simulink model "closeLoopv2"  (R2024a)
settings: Solver=ode4  StartTime=0.0  StopTime=2000  FixedStep=1E-4  MinStep=1E-4  RelTol=1e-3
values from neighbouring files (symbols this model uses):
  initial_1 =     [ma.mat]    (also in regulation.mat)
  x = [input(1);input(2);input(3)]    [Dist_observer.m]    (also in is501nmtbModel_simu.m; is501nmtbModel_simu1.m; ma.mat = ; neuronalPID.m = entr(4))
  y = [input(7),input(8),input(9)]'    [estimator.m]    (also in is501nmtbModel_simu.m = B * x; is501nmtbModel_simu1.m = B * x + Td; ma.mat = ; regulation.mat = )
  z =     [ma.mat]    (also in regulation.mat)
settings Model: Creator=b_ant  LastModifiedBy=b_ant
settings SolverCC: InitialStep=1E-4  ZeroCrossAlgorithm=Adaptive
settings DebuggingCC: IgnoredZcDiagnostic=none

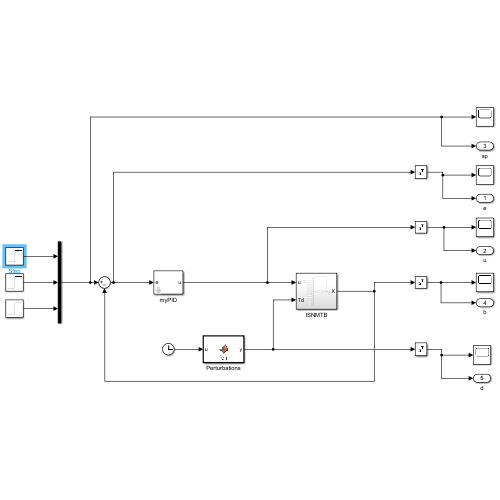
[thumbnail: Simulink's stored preview of the top-level diagram]
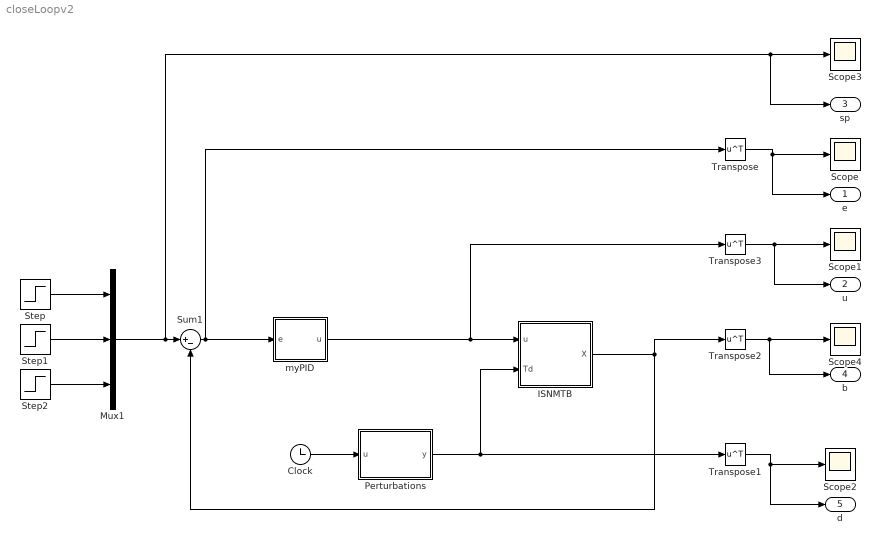
== system closeLoopv2 ==
  Clock : Clock
      settings: Decimation=1000
  ISNMTB : Subsystem
  Mux1 : Mux  Inputs=3
  Perturbations : MATLAB Function  TreatAsAtomicUnit=on
  Scope{,1..4} (5 alike) : Scope
  Step : Step  Time=0.1  After=0  SampleTime=0
  Step1 : Step  Time=0.1  After=0  SampleTime=0
  Step2 : Step  Time=0.1  After=0  SampleTime=0
  Sum1 : Sum  Inputs=|+-
  Transpose{,1..3} (4 alike) : Math  Operator=transpose
  myPID : Subsystem
  e : Outport
  u : Outport  Port=2
  sp : Outport  Port=3
  b : Outport  Port=4
  d : Outport  Port=5
  wires:
  Step2/1 -> Mux1/3
  Sum1/1 -> myPID/1(e), Transpose/1
  Step1/1 -> Mux1/2
  Perturbations/1(y) -> Transpose1/1, ISNMTB/2(Td)
  Clock/1 -> Perturbations/1(u)
  Step/1 -> Mux1/1
  Transpose/1 -> e/1, Scope/1
  Transpose1/1 -> Scope2/1, d/1
  ISNMTB/1(X) -> Transpose2/1, Sum1/2
  Transpose2/1 -> b/1, Scope4/1
  Transpose3/1 -> u/1, Scope1/1
  Mux1/1 -> sp/1, Scope3/1, Sum1/1
  myPID/1(u) -> Transpose3/1, ISNMTB/1(u)

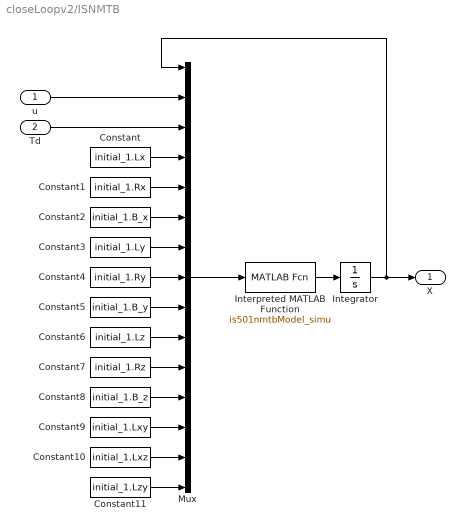
== system closeLoopv2/ISNMTB ==
  u : Inport
  Td : Inport  Port=2
  Constant : Constant  Value=initial_1.Lx
  Constant1 : Constant  Value=initial_1.Rx
  Constant10 : Constant  Value=initial_1.Lxz
  Constant11 : Constant  Value=initial_1.Lzy
  Constant2 : Constant  Value=initial_1.B_x
  Constant3 : Constant  Value=initial_1.Ly
  Constant4 : Constant  Value=initial_1.Ry
  Constant5 : Constant  Value=initial_1.B_y
  Constant6 : Constant  Value=initial_1.Lz
  Constant7 : Constant  Value=initial_1.Rz
  Constant8 : Constant  Value=initial_1.B_z
  Constant9 : Constant  Value=initial_1.Lxy
  Integrator : Integrator  InitialCondition=[3.249E4, -2.265E4, 3.655E4]
  Interpreted MATLAB Function : MATLABFcn  MATLABFcn=is501nmtbModel_simu
  Mux : Mux  Inputs=15
  X : Outport
  wires:
  Interpreted MATLAB Function/1 -> Integrator/1
  Integrator/1 -> X/1, Mux/1
  Mux/1 -> Interpreted MATLAB Function/1
  u/1 -> Mux/2
  Td/1 -> Mux/3
  Constant/1 -> Mux/4
  Constant1/1 -> Mux/5
  Constant2/1 -> Mux/6
  Constant3/1 -> Mux/7
  Constant4/1 -> Mux/8
  Constant5/1 -> Mux/9
  Constant6/1 -> Mux/10
  Constant7/1 -> Mux/11
  Constant8/1 -> Mux/12
  Constant9/1 -> Mux/13
  Constant10/1 -> Mux/14
  Constant11/1 -> Mux/15

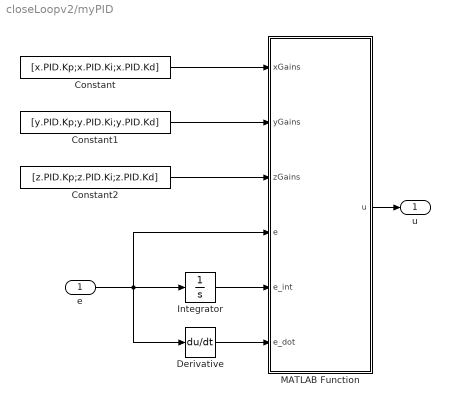
== system closeLoopv2/myPID ==
  e : Inport
  Constant : Constant  Value=[x.PID.Kp;x.PID.Ki;x.PID.Kd]
  Constant1 : Constant  Value=[y.PID.Kp;y.PID.Ki;y.PID.Kd]
  Constant2 : Constant  Value=[z.PID.Kp;z.PID.Ki;z.PID.Kd]
  Derivative : Derivative
  Integrator : Integrator
  MATLAB Function : MATLAB Function  TreatAsAtomicUnit=on
  u : Outport
  wires:
  MATLAB Function/1(u) -> u/1
  e/1 -> Derivative/1, MATLAB Function/4(e), Integrator/1
  Derivative/1 -> MATLAB Function/6(e_dot)
  Integrator/1 -> MATLAB Function/5(e_int)
  Constant1/1 -> MATLAB Function/2(yGains)
  Constant/1 -> MATLAB Function/1(xGains)
  Constant2/1 -> MATLAB Function/3(zGains)

== matlab function closeLoopv2/Perturbations ==
  data: u input; y output
function y = fcn(u)
y= [2.522*sin(2*pi*4.788E-3*u)+3.249E04;
   -5.174*sin(2*pi*7.481E-3*u)-2.265E04;
    3.359*sin(2*pi*8.378E-3*u)+3.655E04];
end

== matlab function closeLoopv2/myPID/MATLAB Function ==
  data: xGains input; u output; yGains input; zGains input; e input; e_int input; e_dot input
function u  = Bpid_controller(xGains, yGains, zGains, e, e_int, e_dot) 
    
    kp = diag([xGains(1),yGains(1),zGains(1)]);
    ki = diag([xGains(2),yGains(2),zGains(2)]);
    kd = diag([xGains(3),yGains(3),zGains(3)]);

    u=kp*e+ki*e_int+kd*e_dot;

end
